simulink model "wheel_steer_estimator_base"  (R2024b)
settings: Solver=FixedStepAuto  StartTime=0.0  StopTime=10.0  RelTol=1e-3
undefined symbols (not defined in the file): mbd_rack_movement, rack_mm, steer_sensor, wheel_steer_left, wheel_steer_right
settings Model: Creator=lukec  LastModifiedBy=lukec
settings OptimizationCC: DefaultParameterBehavior=Inlined  EnhancedBackFolding=on  PassReuseOutputArgsAs=Individual arguments  ZeroExternalMemoryAtStartup=off  ZeroInternalMemoryAtStartup=off  OptimizeBlockOrder=speed  DifferentSizesBufferReuse=on  OptimizationCustomize=off  EfficientTunableParamExpr=on
settings DebuggingCC: ParameterTunabilityLossMsg=error
settings HardwareCC: ProdBitPerPointer=32  ProdBitPerSizeT=32  ProdBitPerPtrDiffT=32  ProdLargestAtomicInteger=Long  ProdLargestAtomicFloat=Double  ProdWordSize=32  ProdHWDeviceType=ARM Compatible->ARM Cortex-M
settings SFSimCC: MATLABDynamicMemAlloc=off
settings RTWCC: Description=Embedded Coder  SystemTargetFile=ert.tlc  GenCodeOnly=on  PackageGeneratedCodeAndArtifacts=on  TemplateMakefile=ert_default_tmf  Toolchain=CMake  TargetLang=C++  HalideCodeGeneration=on
settings CodeAppCC: ForceParamTrailComments=on  IgnoreCustomStorageClasses=off  MaxIdLength=255  OperatorAnnotations=on  SimulinkDataObjDesc=on  SFDataObjDesc=on  InsertBlockDesc=on
settings ERTTargetCC: TargetLangStandard=C++17 (ISO)  CodeInterfacePackaging=C++ class  RootIOFormat=Structure reference  ERTCustomFileTemplate=example_file_process.tlc  ArrayContainerType=std::array

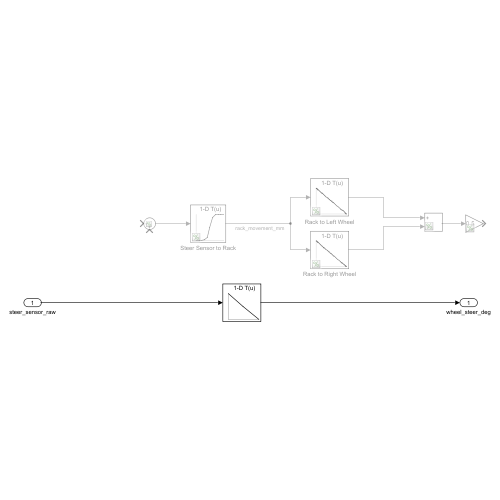
[thumbnail: Simulink's stored preview of the top-level diagram]
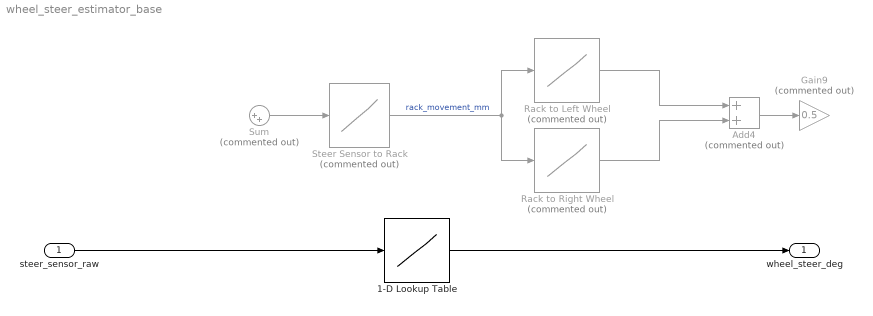
== system wheel_steer_estimator_base ==
  steer_sensor_raw : Inport
  1-D Lookup Table : Lookup_n-D  NumberOfTableDimensions=1  BreakpointsForDimension1=[211 1129 2133]  Table=[23 0 -23]  ExtrapMethod=Clip  UseLastTableValue=on  InternalRulePriority=Speed  RndMeth=Simplest
  Add4 : Sum  Commented=on
  Gain9 : Gain  Commented=on  Gain=0.5
  Rack to Left Wheel : Lookup_n-D  Commented=on  NumberOfTableDimensions=1  BreakpointsForDimension1=mbd_rack_movement  Table=wheel_steer_left  ExtrapMethod=Clip  UseLastTableValue=on  InternalRulePriority=Speed  RndMeth=Simplest
  Rack to Right Wheel : Lookup_n-D  Commented=on  NumberOfTableDimensions=1  BreakpointsForDimension1=mbd_rack_movement  Table=wheel_steer_right  ExtrapMethod=Clip  UseLastTableValue=on  InternalRulePriority=Speed  RndMeth=Simplest
  Steer Sensor to Rack : Lookup_n-D  Commented=on  NumberOfTableDimensions=1  LookupTableObject=PLEASE  BreakpointsForDimension1=steer_sensor  Table=rack_mm  ExtrapMethod=Clip  InternalRulePriority=Speed  RndMeth=Simplest
  Sum : Sum  Commented=on  Inputs=|++
  wheel_steer_deg : Outport
  wires:
  Rack to Right Wheel/1 -> Add4/2
  Steer Sensor to Rack/1 -> Rack to Left Wheel/1, Rack to Right Wheel/1  "rack_movement_mm"
  Add4/1 -> Gain9/1
  Sum/1 -> Steer Sensor to Rack/1
  Rack to Left Wheel/1 -> Add4/1
  steer_sensor_raw/1 -> 1-D Lookup Table/1
  1-D Lookup Table/1 -> wheel_steer_deg/1
